simulink model "Wheelspeed_Logik_First_code_Mdian_try"  (R2025b)
settings: Solver=ode1  StartTime=0.0  StopTime=10.0  FixedStep=0.0001  RelTol=1e-3
libraries: simulink x2
settings Model: Creator=finneinhoff  LastModifiedBy=finneinhoff

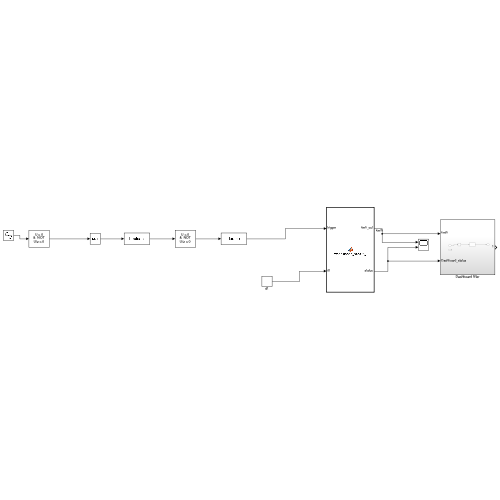
[thumbnail: Simulink's stored preview of the top-level diagram]
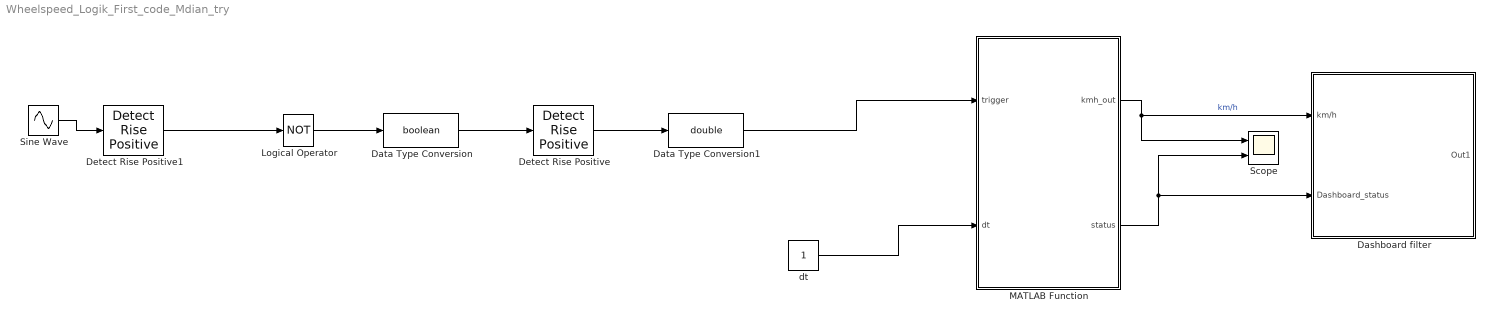
== system Wheelspeed_Logik_First_code_Mdian_try ==
  Dashboard filter : Subsystem
  Data Type Conversion : DataTypeConversion  OutDataTypeStr=boolean  SaturateOnIntegerOverflow=off  RndMeth=Floor
  Data Type Conversion1 : DataTypeConversion  OutDataTypeStr=double  SaturateOnIntegerOverflow=off  RndMeth=Floor
  Detect Rise Positive : simulink/Logic and Bit Operations/Detect Rise Positive  vinit=0  OutDataTypeStr=boolean
  Detect Rise Positive1 : simulink/Logic and Bit Operations/Detect Rise Positive  vinit=0  OutDataTypeStr=boolean
  Logical Operator : Logic  Operator=NOT  AllPortsSameDT=off  OutDataTypeStr=boolean
  MATLAB Function : MATLAB Function  TreatAsAtomicUnit=on
  Scope : Scope  NumInputPorts=2
      settings: ActiveDisplayYMinimum=27.946667618257287  ActiveDisplayYMaximum=31.262681766179149
  Sine Wave : Sin  SampleTime=0
  dt : Constant
  wires:
  Logical Operator/1 -> Data Type Conversion/1
  Detect Rise Positive/1 -> Data Type Conversion1/1
  MATLAB Function/1(kmh_out) -> Scope/1, Dashboard filter/1(km/h)  "km/h"
  Data Type Conversion/1 -> Detect Rise Positive/1
  Sine Wave/1 -> Detect Rise Positive1/1
  Detect Rise Positive1/1 -> Logical Operator/1
  Data Type Conversion1/1 -> MATLAB Function/1(trigger)
  dt/1 -> MATLAB Function/2(dt)
  MATLAB Function/2(status) -> Dashboard filter/2(Dashboard_status), Scope/2

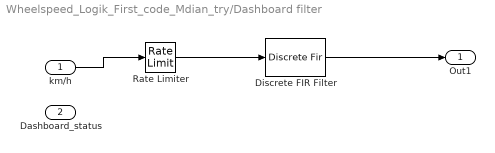
== system Wheelspeed_Logik_First_code_Mdian_try/Dashboard filter ==
  km/h : Inport
  Dashboard_status : Inport  Port=2
  Discrete FIR Filter : DiscreteFir
  Rate Limiter : RateLimiter  SampleTimeMode=inherited
  Out1 : Outport
  wires:
  km/h/1 -> Rate Limiter/1
  Rate Limiter/1 -> Discrete FIR Filter/1
  Discrete FIR Filter/1 -> Out1/1

== matlab function Wheelspeed_Logik_First_code_Mdian_try/MATLAB Function ==
  data: trigger input; kmh_out output; dt input; status output
function [kmh_out, status] = wheelspeed_fs2026_(trigger, dt)
    
    teeth = 50;
    circum = 1.6;
    
    
    % Grenzen
    MIN_SPEED_KMH = 3.0;       
    MAX_ACCEL_G   = 4.5;       
    
    % Filter-Dynamik (Gemini)
    ALPHA_STEADY  = 0.15;      % Sehr glatt beim Cruisen (starke Filterung)
    ALPHA_AGILE   = 0.90;      % Fast ungefiltert bei Wheelspin (geringe Latenz)
    ACCEL_THRESH  = 1.5;       % Ab 1.5G Beschleunigung schaltet der Filter auf "Agil"
    
    % Speicher
    persistent timer;           % Exakter Timer
    persistent raw_buffer;      % Buffer für Median-Filter (3 werte)
    persistent v_smooth;        % geglätteter Output
    persistent last_period;     % Für Plausibilitätsprüfung
    persistent first_run;       % Initialisierung
    
    % Kaltstart
    if isempty(timer)
        timer = 0;
        raw_buffer = [0.1, 0.1, 0.1]; % 3 Dummy werte
        v_smooth = 0;
        last_period = 0.1;
        first_run = true;
    end
    
    % 1. TIMER update
    timer = timer + dt;
    status = 0; % Default: Warten
    
    % trigger
    if trigger >= 1
        current_period = timer;
        
        
        %theoretische Geschwindigkeit 1 Puls
        dist_per_tooth = circum / teeth;
        v_inst_raw_ms = dist_per_tooth / current_period;
        
        % Plausubilitätsprüfung
        
        current_v_ms = v_smooth / 3.6;
        
        % theoretische Beschleunigung
        inst_accel = (v_inst_raw_ms - current_v_ms) / current_period;
        
        % ok bei anfahren oder wenn plausibel
        if (abs(inst_accel) < (MAX_ACCEL_G * 9.81)) || (v_inst_raw_ms < 2.0)
            
            % Median-Filter
            raw_buffer(1) = raw_buffer(2);
            raw_buffer(2) = raw_buffer(3);
            raw_buffer(3) = current_period;
            
            % Berechne Median 3 Werte
            p1 = raw_buffer(1); p2 = raw_buffer(2); p3 = raw_buffer(3);
            if p1 > p2; tmp=p1; p1=p2; p2=tmp; end
            if p2 > p3; tmp=p2; p2=p3; p3=tmp; end
            if p1 > p2; p1=p2; end % p2  jetzt Median
            clean_period = p2;
            
            % geschw.
            v_inst_clean_ms = dist_per_tooth / clean_period;
            
            % trend
            trend = v_inst_clean_ms - (v_smooth / 3.6);
            
            % Gemini
            if trend > 0 
                % POSITIVE Flanke (Beschleunigung/Wheelspin): 
                % Wir wollen null Latenz! Filter öffnen!
                % Wir mappen die Beschleunigung auf Alpha.
                % Je stärker der Wheelspin, desto "roher" das Signal.
                accel_factor = min(abs(trend) / (ACCEL_THRESH * 9.81 * current_period), 1.0);
                alpha = ALPHA_STEADY + (ALPHA_AGILE - ALPHA_STEADY) * accel_factor;
            else
                % NEGATIVE Flanke (Bremsen/Ausrollen) oder Konstante Fahrt:
                % Wir wollen maximales Glätten gegen Vibrationen.
                alpha = ALPHA_STEADY;
            end
            
            % Filter anwenden (EMA)
            % v_neu = alpha * raw + (1-alpha) * alt
            v_new_ms = alpha * v_inst_clean_ms + (1-alpha) * (v_smooth / 3.6);
            
            % Output
            v_smooth = v_new_ms * 3.6;
            last_period = clean_period;
            status = 1; % Valid update
            
            % Timer reset 
            timer = 0;
            first_run = false;
        else
            status = 2; % Rejected
        end
    end
    
    
    % estimate nächster zahn time
    if v_smooth > MIN_SPEED_KMH
        v_ms = v_smooth / 3.6;
        expected_period = (circum / teeth) / v_ms;
        
        % wenn wir zu lange warten
        if timer > (expected_period * 2.0)
        end
    end
    
    % stillstand
    if (timer > 0.5)
        v_smooth = 0;
        status = 3;% Stillstand
    end
    
    % Output
    kmh_out = v_smooth;
end
